simulink model "downcount_test"  (R2019b)
settings: Solver=FixedStepDiscrete  StartTime=0.0  StopTime=100  RelTol=1e-3
libraries: simulink x1, lib_dsphdlcontrol_v1 x1
settings Model: DataTypeOverride=Off  Creator=mbabst  LastModifiedBy=mbabst
settings DataIOCC: SaveOutput=off  SaveTime=off  ReturnWorkspaceOutputs=off
settings OptimizationCC: BlockReduction=off  ConditionallyExecuteInputs=off  DefaultParameterBehavior=Inlined  LifeSpan=inf
settings DebuggingCC: AlgebraicLoopMsg=error  SingleTaskRateTransMsg=error  StrictBusMsg=ErrorOnBusTreatedAsVector  SFUnexpectedBacktrackingDiag=warning  SFNoUnconditionalDefaultTransitionDiag=warning  ArithmeticOperatorsInVariantConditions=warning
settings HardwareCC: ProdBitPerPointer=32  ProdBitPerSizeT=32  ProdBitPerPtrDiffT=32  ProdLargestAtomicFloat=None  ProdIntDivRoundTo=Undefined  ProdEndianess=Unspecified  ProdWordSize=32  ProdHWDeviceType=ASIC/FPGA->ASIC/FPGA  ProdEqTarget=off
settings SFSimCC: SimUseLocalCustomCode=off  CustomCodeUndefinedFunction=UseInterfaceOnly
settings RTWCC: RTWUseLocalCustomCode=off
settings CodeAppCC: StateflowObjectComments=on
settings GRTTargetCC: TargetLangStandard=C89/C90 (ANSI)  GeneratePreprocessorConditionals=Disable all
settings ConfigComp: CovMetricSettings=dw  CovHtmlReporting=on  CovSaveCumulativeToWorkspaceVar=on  CovSaveSingleToWorkspaceVar=on  CovExternalEMLEnable=off

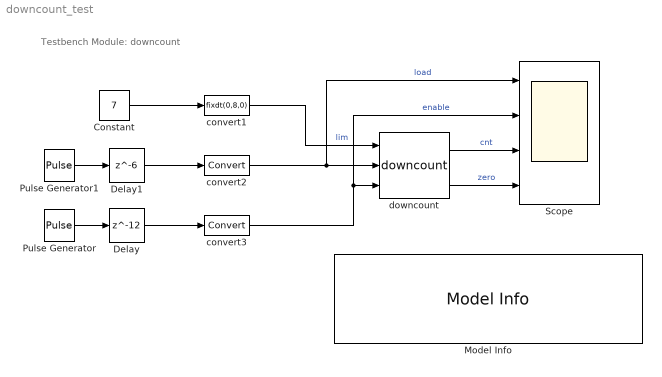
== system downcount_test ==
  note: Testbench
      | Module: downcount
  Constant : Constant  Value=7
  Delay : Delay  DelayLength=12  InitialCondition=0
  Delay1 : Delay  DelayLength=6  InitialCondition=0
  Model Info : simulink/Model-Wide Utilities/Model Info  Frame=on  DisplayStringWithTags=|  HorizontalTextAlignment=Left  LeftAlignmentValue=0.02
      | Copyright (c) 2005-2021 DSPlogic, Inc.
      | Distributed under the terms of the Simplified BSD License.
      | The full license is in the file LICENSE, distributed with this software.
      | 
      | Model: %<ModelName> (v%<ModelVersion>)
      | Author: Michael Babst <mike.babst@dsplogic.com>
      | Created: by %<Creator> on %<Created>
      | Modified: by %<ModifiedBy> on %<LastModificationDate>
  Pulse Generator : DiscretePulseGenerator  Period=3  PulseWidth=3
  Pulse Generator1 : DiscretePulseGenerator  Period=50  PhaseDelay=2
  Scope : Scope  NumInputPorts=4
  convert1 : DataTypeConversion  OutDataTypeStr=fixdt(0,8,0)
  convert2 : DataTypeConversion
  convert3 : DataTypeConversion
  downcount : lib_dsphdlcontrol_v1/downcount  FreeRun=on
      settings: SourceProductName=DSPHDL Library
  wires:
  Pulse Generator1/1 -> Delay1/1
  Pulse Generator/1 -> Delay/1
  Constant/1 -> convert1/1
  downcount/1 -> Scope/3  "cnt"
  downcount/2 -> Scope/4  "zero"
  convert1/1 -> downcount/1  "lim"
  convert2/1 -> downcount/2, Scope/1  "load"
  Delay/1 -> convert3/1
  convert3/1 -> downcount/3, Scope/2  "enable"
  Delay1/1 -> convert2/1
